simulink subsystem "Fuzzy_PI_Controller"  (R2023a)
settings: Solver=VariableStepAuto  StartTime=0.0  StopTime=10.0  RelTol=1e-3
libraries: fuzblock x1
settings Model: Creator=Νίκος  LastModifiedBy=Νίκος

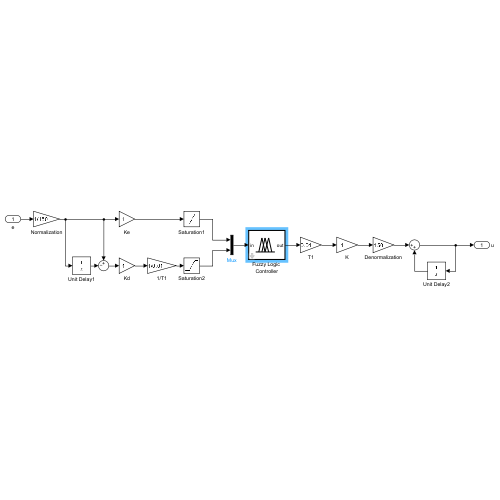
[thumbnail: Simulink's stored preview of the top-level diagram]
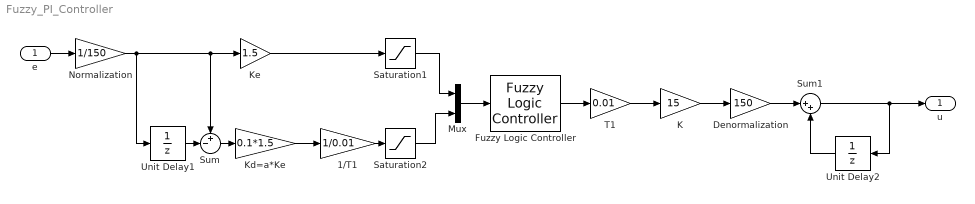
== system Fuzzy_PI_Controller ==
  e : Inport
  1/T1 : Gain  Gain=1/0.01
  Denormalization : Gain  Gain=150
  Fuzzy Logic Controller : fuzblock/Fuzzy Logic  Controller  FIS='Fuzzy_Controller.fis'  OutputSampleNumber=101  DataType=double  FuzzifiedInputs=off  RuleFiringStrengths=off  RuleOutputs=off  AggregatedOutputs=off  SimulateUsing=Interpreted execution  OutOfRangeInputValueMessage=warning  NoRuleFiredMessage=warning  EmptyOutputFuzzySetMessage=warning
  K : Gain  Gain=15
  Kd=a*Ke : Gain  Gain=0.1*1.5
  Ke : Gain  Gain=1.5
  Mux : Mux  Inputs=2
  Normalization : Gain  Gain=1/150
  Saturation1 : Saturate
  Saturation2 : Saturate
  Sum : Sum  Inputs=+-|
  Sum1 : Sum  Inputs=|++
  T1 : Gain  Gain=0.01
  Unit Delay1 : UnitDelay  SampleTime=-1  HasFrameUpgradeWarning=on
  Unit Delay2 : UnitDelay  SampleTime=-1  HasFrameUpgradeWarning=on
  u : Outport  SignalName=u
  wires:
  e/1 -> Normalization/1
  Normalization/1 -> Ke/1, Sum/1, Unit Delay1/1
  Unit Delay1/1 -> Sum/2
  Sum/1 -> Kd=a*Ke/1
  Kd=a*Ke/1 -> 1/T1/1
  1/T1/1 -> Saturation2/1
  Ke/1 -> Saturation1/1
  Saturation1/1 -> Mux/1
  Saturation2/1 -> Mux/2
  Mux/1 -> Fuzzy Logic Controller/1
  Fuzzy Logic Controller/1 -> T1/1
  T1/1 -> K/1
  K/1 -> Denormalization/1
  Sum1/1 -> Unit Delay2/1, u/1
  Denormalization/1 -> Sum1/1
  Unit Delay2/1 -> Sum1/2
